simulink model "SRM_Drive_Model"  (R2024a)
settings: Solver=VariableStepAuto  StartTime=0.0  StopTime=2  RelTol=1e-3
undefined symbols (not defined in the file): DiscIntNeverNeededParam
libraries: spsDiodeLib x6, spsIGBTLib x6, spsDCVoltageSourceLib x1, spsSwitchedReluctanceMotorLib x1, spspowerguiLib x1
settings Model: Creator=richa  LastModifiedBy=richa

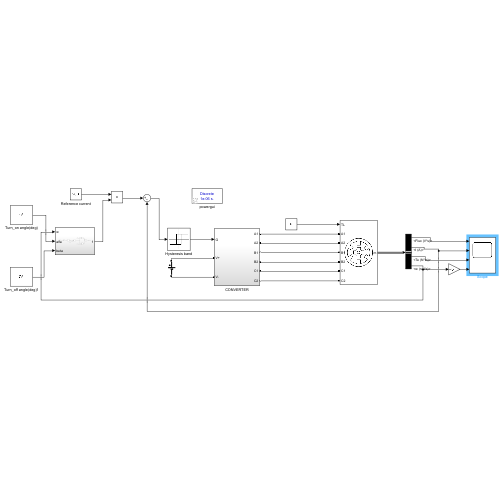
[thumbnail: Simulink's stored preview of the top-level diagram]
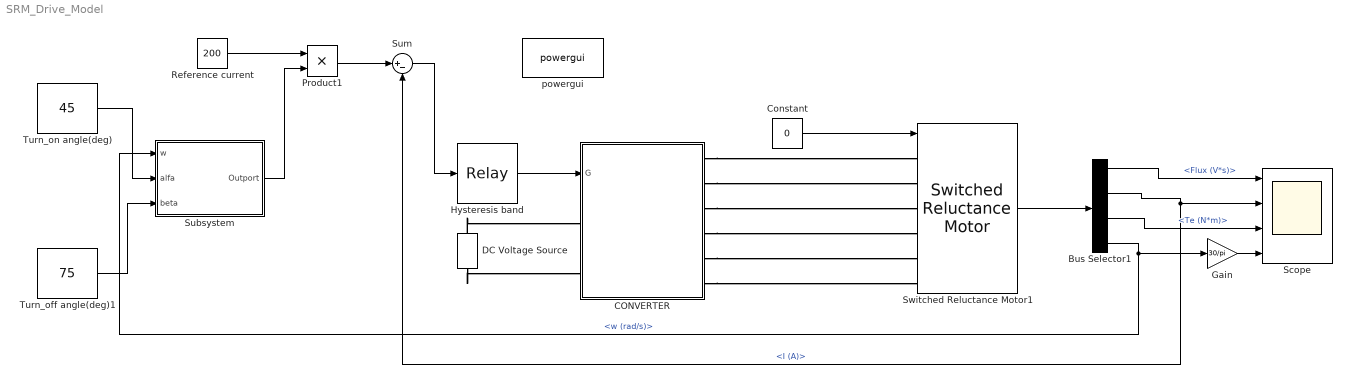
== system SRM_Drive_Model ==
  Bus Selector1 : BusSelector  OutputSignals=Flux (V*s),I (A),Te (N*m),w (rad/s)
  CONVERTER : Subsystem
  Constant : Constant  Value=0
  DC Voltage Source : spsDCVoltageSourceLib/DC Voltage Source  Amplitude=240  Measurements=None
  Gain : Gain  Gain=30/pi
  Hysteresis band : Relay  OnSwitchValue=10  OffSwitchValue=-10
  Product1 : Product
  Reference current : Constant  Value=200
  Scope : Scope  NumInputPorts=4
  Subsystem : Subsystem
  Sum : Sum  Inputs=|+-
  Switched Reluctance Motor1 : spsSwitchedReluctanceMotorLib/Switched Reluctance Motor  MachineType=6/4  StatorResistance=0.05  Inertia=0.05  Friction=0.02  InitialSpeed=[0 0]  TsPowergui=0  TsBlock=5e-6  MachineModel=Specific model  Lq=0.67e-3  Ld=23.6e-3  Lsat=0.15e-3  MaximumCurrent=450  MaximumFluxLinkage=0.486  Source=MAT-file  MagnetisationCharacteristic='srm64_60kw.mat'  RotorAngleVector=[0 10 20 30 40 45]  StatorCurrentVector=[0:25:450]  PlotCurves=off
      settings: LibrarySourceBlock=|
      | sps_lib/Electrical Machines/Switched Reluctance
      | Motor
  Turn_off angle(deg)1 : Constant  Value=75
  Turn_on angle(deg) : Constant  Value=45
  powergui : spspowerguiLib/powergui  Priority=1  SimulationMode=Discrete  SampleTime=1e-06  frequency=60  Iterations=50  frequencyindice=0  Pbase=100e6  ErrMax=1e-4  UnitsV=kV  UnitsW=MW  buscounter=0  FunctionMessages=off  echomessages=off  EnableUseOfTLC=off  CurrentSourceSwitches=off  DisableSnubberDevices=off  DisableRonSwitches=off  DisableVfSwitches=off  DisplayEquations=off  AutomaticDiscreteSolvers=off  SolverType=Tustin/Backward Euler (TBE)  Interpol=off  ExternalGateDelay=off  methode=off  Ts=100  x0status=blocks  SPID=on  SwTol=0  HookPort=off  NonlinearTolerance=1e-4  nMaxIteration=100  ContinueOnMaxIteration=off  RestoreLinks=warning  ResistiveCurrentMeasurement=off  Frange=[0:2:500]  Ylog=off  Xlog=on  ShowGrid=off  save=off  variable=ZData  structure=0  ZoomFFT=off  StartTime=0.0  cycles=1  DisplayStyle=1  fundamental=60  FreqAxis=off  MaxFrequency=1000  frequencyindicesteady=1  RmsSteady=1  display=off
  wires:
  Constant/1 -> Switched Reluctance Motor1/1
  Hysteresis band/1 -> CONVERTER/1(G)
  Switched Reluctance Motor1/1 -> Bus Selector1/1
  Bus Selector1/1 -> Scope/1  "<Flux (V*s)>"
  Bus Selector1/2 -> Scope/2, Sum/2  "<I (A)>"
  Bus Selector1/3 -> Scope/3  "<Te (N*m)>"
  Bus Selector1/4 -> Subsystem/1(w), Gain/1  "<w (rad/s)>"
  Reference current/1 -> Product1/1
  Turn_on angle(deg)/1 -> Subsystem/2(alfa)
  Turn_off angle(deg)1/1 -> Subsystem/3(beta)
  Subsystem/1(Outport) -> Product1/2
  Product1/1 -> Sum/1
  Sum/1 -> Hysteresis band/1
  Gain/1 -> Scope/4
  connections:
  CONVERTER/RConn4 -- Switched Reluctance Motor1/LConn4
  CONVERTER/RConn5 -- Switched Reluctance Motor1/LConn5
  CONVERTER/RConn6 -- Switched Reluctance Motor1/LConn6
  CONVERTER/RConn3 -- Switched Reluctance Motor1/LConn3
  CONVERTER/RConn2 -- Switched Reluctance Motor1/LConn2
  CONVERTER/RConn1 -- Switched Reluctance Motor1/LConn1
  DC Voltage Source/RConn1 -- CONVERTER/LConn1
  DC Voltage Source/LConn1 -- CONVERTER/LConn2

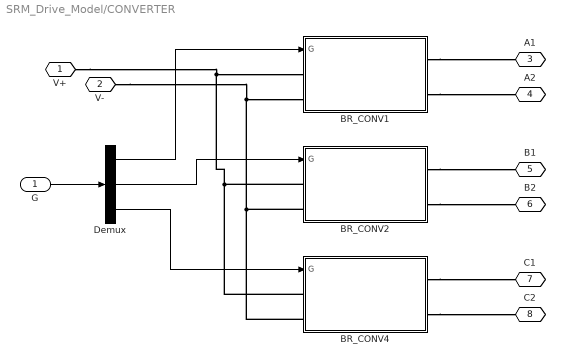
== system SRM_Drive_Model/CONVERTER ==
  G : Inport
  BR_CONV1 : Subsystem
  BR_CONV2 : Subsystem
  BR_CONV4 : Subsystem
  Demux : Demux  Outputs=3
  V+ : PMIOPort  Side=Left
  V- : PMIOPort  Port=2  Side=Left
  A1 : PMIOPort  Port=3  Side=Right
  A2 : PMIOPort  Port=4  Side=Right
  B1 : PMIOPort  Port=5  Side=Right
  B2 : PMIOPort  Port=6  Side=Right
  C1 : PMIOPort  Port=7  Side=Right
  C2 : PMIOPort  Port=8  Side=Right
  wires:
  G/1 -> Demux/1
  Demux/1 -> BR_CONV1/1(G)
  Demux/2 -> BR_CONV2/1(G)
  Demux/3 -> BR_CONV4/1(G)
  connections:
  V+/RConn1 -- BR_CONV4/LConn1 -- BR_CONV2/LConn1 -- BR_CONV1/LConn1
  V-/RConn1 -- BR_CONV2/LConn2 -- BR_CONV4/LConn2 -- BR_CONV1/LConn2
  BR_CONV1/RConn1 -- A1/RConn1
  BR_CONV1/RConn2 -- A2/RConn1
  BR_CONV2/RConn1 -- B1/RConn1
  BR_CONV2/RConn2 -- B2/RConn1
  BR_CONV4/RConn1 -- C1/RConn1
  BR_CONV4/RConn2 -- C2/RConn1

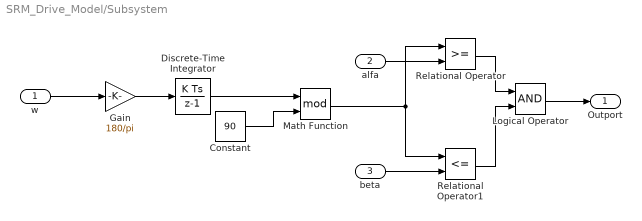
== system SRM_Drive_Model/Subsystem ==
  w : Inport
  alfa : Inport  Port=2
  beta : Inport  Port=3
  Constant : Constant  Value=90
  Discrete-Time Integrator : DiscreteIntegrator  InitialCondition=[0 -30 -60]  SampleTime=-1  ICPrevOutput=DiscIntNeverNeededParam  ICPrevScaledInput=DiscIntNeverNeededParam
  Gain : Gain  Gain=180/pi
  Logical Operator : Logic  AllPortsSameDT=off  OutDataTypeStr=boolean
  Math Function : Math  Operator=mod
  Relational Operator : RelationalOperator  OutDataTypeStr=boolean  RndMeth=Simplest  InputSameDT=off
  Relational Operator1 : RelationalOperator  Operator=<=  OutDataTypeStr=boolean  RndMeth=Simplest  InputSameDT=off
  Outport : Outport
  wires:
  w/1 -> Gain/1
  Gain/1 -> Discrete-Time Integrator/1
  Discrete-Time Integrator/1 -> Math Function/1
  Constant/1 -> Math Function/2
  Math Function/1 -> Relational Operator/1, Relational Operator1/1
  alfa/1 -> Relational Operator/2
  beta/1 -> Relational Operator1/2
  Relational Operator/1 -> Logical Operator/1
  Relational Operator1/1 -> Logical Operator/2
  Logical Operator/1 -> Outport/1

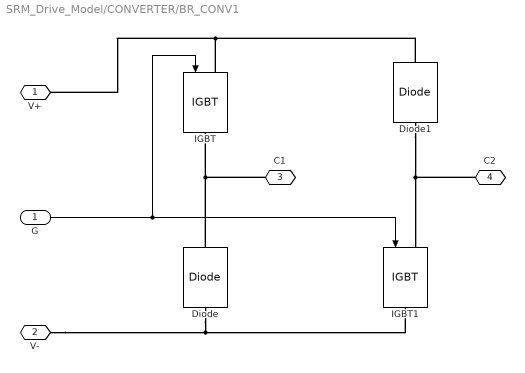
== system SRM_Drive_Model/CONVERTER/BR_CONV1 ==
  G : Inport
  Diode : spsDiodeLib/Diode  Ron=1E-3  Lon=0  Vf=0.8  IC=0  UseSnubber=0  Rs=1000  Cs=inf  Measurements=off
  Diode1 : spsDiodeLib/Diode  Ron=1E-3  Lon=0  Vf=0.8  IC=0  UseSnubber=0  Rs=1000  Cs=inf  Measurements=off
  IGBT : spsIGBTLib/IGBT  Ron=1e-3  Lon=0  Vf=1  Tf=1e-6  Tt=2e-6  IC=0  Rs=200  Cs=0.1E-06  Measurements=off
  IGBT1 : spsIGBTLib/IGBT  Ron=1e-3  Lon=0  Vf=1  Tf=1e-6  Tt=2e-6  IC=0  Rs=200  Cs=0.1E-06  Measurements=off
  V+ : PMIOPort  Side=Left
  V- : PMIOPort  Port=2  Side=Left
  C1 : PMIOPort  Port=3  Side=Right
  C2 : PMIOPort  Port=4  Side=Right
  wires:
  G/1 -> IGBT/1, IGBT1/1
  connections:
  Diode1/RConn1 -- IGBT/LConn1 -- V+/RConn1
  Diode/RConn1 -- C1/RConn1 -- IGBT/RConn1
  Diode1/LConn1 -- C2/RConn1 -- IGBT1/LConn1
  V-/RConn1 -- Diode/LConn1 -- IGBT1/RConn1

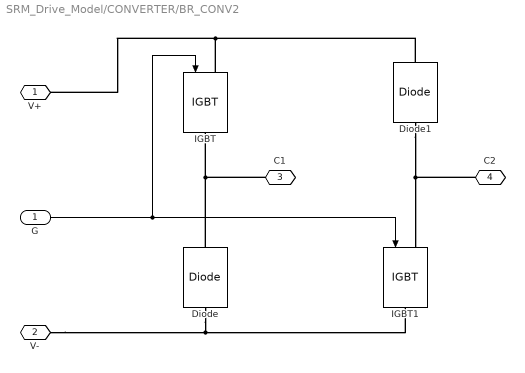
== system SRM_Drive_Model/CONVERTER/BR_CONV2 ==
  G : Inport
  Diode : spsDiodeLib/Diode  Ron=1E-3  Lon=0  Vf=0.8  IC=0  UseSnubber=0  Rs=1000  Cs=inf  Measurements=off
  Diode1 : spsDiodeLib/Diode  Ron=1E-3  Lon=0  Vf=0.8  IC=0  UseSnubber=0  Rs=1000  Cs=inf  Measurements=off
  IGBT : spsIGBTLib/IGBT  Ron=1e-3  Lon=0  Vf=1  Tf=1e-6  Tt=2e-6  IC=0  Rs=200  Cs=0.1E-06  Measurements=off
  IGBT1 : spsIGBTLib/IGBT  Ron=1e-3  Lon=0  Vf=1  Tf=1e-6  Tt=2e-6  IC=0  Rs=200  Cs=0.1E-06  Measurements=off
  V+ : PMIOPort  Side=Left
  V- : PMIOPort  Port=2  Side=Left
  C1 : PMIOPort  Port=3  Side=Right
  C2 : PMIOPort  Port=4  Side=Right
  wires:
  G/1 -> IGBT1/1, IGBT/1
  connections:
  Diode/LConn1 -- V-/RConn1 -- IGBT1/RConn1
  C2/RConn1 -- Diode1/LConn1 -- IGBT1/LConn1
  C1/RConn1 -- Diode/RConn1 -- IGBT/RConn1
  IGBT/LConn1 -- V+/RConn1 -- Diode1/RConn1

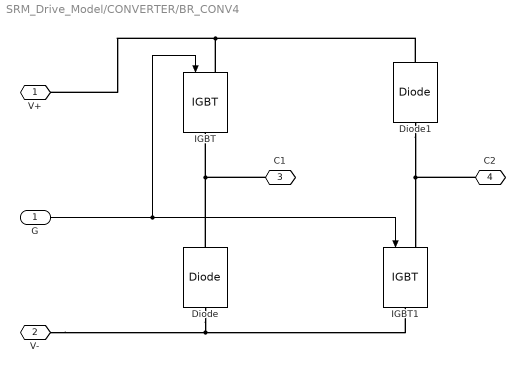
== system SRM_Drive_Model/CONVERTER/BR_CONV4 ==
  G : Inport
  Diode : spsDiodeLib/Diode  Ron=1E-3  Lon=0  Vf=0.8  IC=0  UseSnubber=0  Rs=1000  Cs=inf  Measurements=off
  Diode1 : spsDiodeLib/Diode  Ron=1E-3  Lon=0  Vf=0.8  IC=0  UseSnubber=0  Rs=1000  Cs=inf  Measurements=off
  IGBT : spsIGBTLib/IGBT  Ron=1e-3  Lon=0  Vf=1  Tf=1e-6  Tt=2e-6  IC=0  Rs=200  Cs=0.1E-06  Measurements=off
  IGBT1 : spsIGBTLib/IGBT  Ron=1e-3  Lon=0  Vf=1  Tf=1e-6  Tt=2e-6  IC=0  Rs=200  Cs=0.1E-06  Measurements=off
  V+ : PMIOPort  Side=Left
  V- : PMIOPort  Port=2  Side=Left
  C1 : PMIOPort  Port=3  Side=Right
  C2 : PMIOPort  Port=4  Side=Right
  wires:
  G/1 -> IGBT1/1, IGBT/1
  connections:
  Diode/LConn1 -- V-/RConn1 -- IGBT1/RConn1
  C2/RConn1 -- Diode1/LConn1 -- IGBT1/LConn1
  C1/RConn1 -- Diode/RConn1 -- IGBT/RConn1
  IGBT/LConn1 -- V+/RConn1 -- Diode1/RConn1
